simulink model "Q2_t"  (R2021b)
settings: Solver=VariableStepAuto  StartTime=0.0  StopTime=20  RelTol=1e-3
settings Model: Creator=nima8  LastModifiedBy=nima8

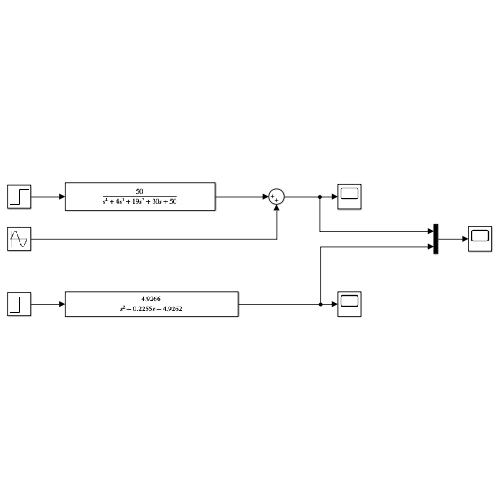
[thumbnail: Simulink's stored preview of the top-level diagram]
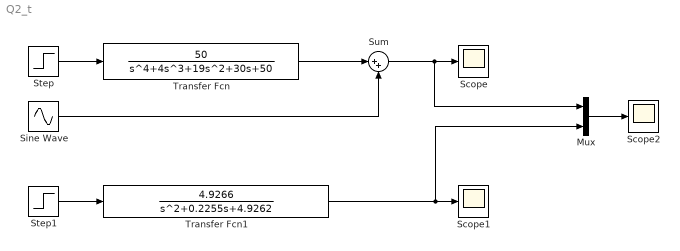
== system Q2_t ==
  Mux : Mux  Inputs=2
  Scope : Scope
  Scope1 : Scope
  Scope2 : Scope
  Sine Wave : Sin  Amplitude=0.05  Frequency=40  SampleTime=0
  Step : Step  Time=0  SampleTime=0
  Step1 : Step  Time=0  SampleTime=0
  Sum : Sum  Inputs=|++
  Transfer Fcn : TransferFcn  Numerator=[50]  Denominator=[1 4 19 30 50]
  Transfer Fcn1 : TransferFcn  Numerator=[4.9266]  Denominator=[1 0.2255 4.9262]
  wires:
  Step/1 -> Transfer Fcn/1
  Transfer Fcn/1 -> Sum/1
  Sum/1 -> Mux/1, Scope/1
  Sine Wave/1 -> Sum/2
  Transfer Fcn1/1 -> Mux/2, Scope1/1
  Step1/1 -> Transfer Fcn1/1
  Mux/1 -> Scope2/1
